simulink model "FixedWing"  (R2024b)
settings: Solver=VariableStepAuto  StartTime=0.0  StopTime=10.0  RelTol=1e-3
undefined symbols (not defined in the file): AirSpeed, Height, RollAngle
libraries: simulink_extras x3, uavalgslib x1
settings Model: Creator=shiva  LastModifiedBy=shiva

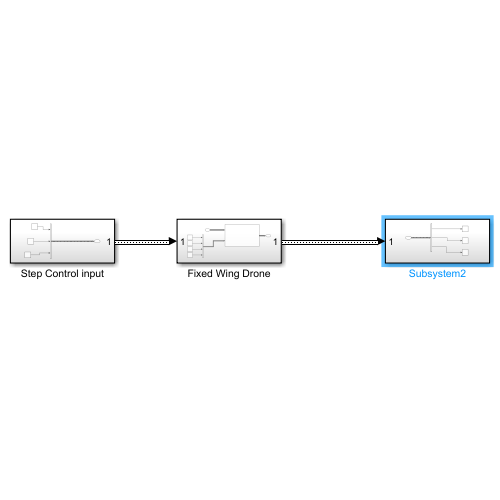
[thumbnail: Simulink's stored preview of the top-level diagram]
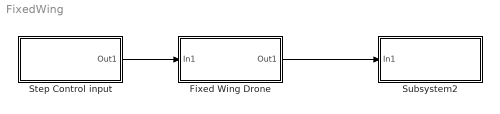
== system FixedWing ==
  Fixed Wing Drone : Subsystem
  Step Control input : Subsystem
  Subsystem2 : Subsystem
  wires:
  Step Control input/1(Out1) -> Fixed Wing Drone/1(In1)
  Fixed Wing Drone/1(Out1) -> Subsystem2/1(In1)

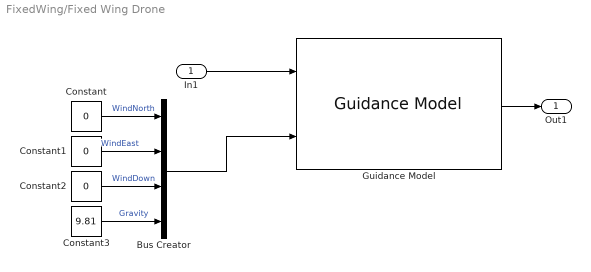
== system FixedWing/Fixed Wing Drone ==
  In1 : Inport
  Bus Creator : BusCreator  Inputs=4  OutDataTypeStr=Bus: FixedWingGuidanceEnvironmentBus  NonVirtualBus=on
  Constant : Constant  Value=0
  Constant1 : Constant  Value=0
  Constant2 : Constant  Value=0
  Constant3 : Constant  Value=9.81
  Guidance Model : uavalgslib/Guidance Model  ModelType=FixedWingGuidance  SpecifiedDataType=double  SimulateUsing=Interpreted execution  InitialWorldPositionMultirotor=[0; 0; 0]  InitialWorldVelocityMultirotor=[0; 0; 0]  InitialEulerZYXMultirotor=[0; 0; 0]  InitialBodyAngularRateRPYMultirotor=[0; 0; 0]  InitialThrustMultirotor=0  InitialNorthFixedWing=0  InitialEastFixedWing=0  InitialHeightFixedWing=0  InitialAirSpeedFixedWing=0  InitialHeadingAngleFixedWing=0  InitialFlightPathAngleFixedWing=0  InitialRollAngleFixedWing=0  InitialRollAngleRateFixedWing=0  PDRollMultirotor=[3402.97,116.67]  PDPitchMultirotor=[3402.97, 116.67]  PYawRateMultirotor=1950  PThrustMultirotor=3900  MassMultirotor=0.1  PHeightFixedWing=3.9  PHeadingAngleFixedWing=3.9  PFlightPathAngleFixedWing=39  PDRollFixedWing=[3402.97, 116.67]  PAirSpeedFixedWing=1  FlightPathAngleLimitsFixedWing=[-pi/2, pi/2]  StateBusName='FixedWingGuidanceStateBus'  ControlBusName='FixedWingGuidanceControlBus'  EnvironmentBusName='FixedWingGuidanceEnvironmentBus'  DataType=double
  Out1 : Outport
  wires:
  Guidance Model/1 -> Out1/1
  In1/1 -> Guidance Model/1
  Bus Creator/1 -> Guidance Model/2
  Constant/1 -> Bus Creator/1  "WindNorth"
  Constant1/1 -> Bus Creator/2  "WindEast"
  Constant2/1 -> Bus Creator/3  "WindDown"
  Constant3/1 -> Bus Creator/4  "Gravity"

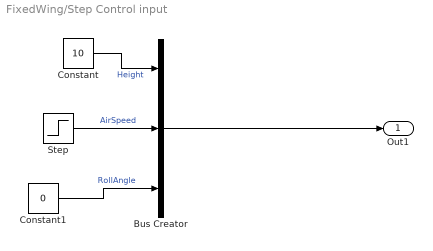
== system FixedWing/Step Control input ==
  Bus Creator : BusCreator  Inputs=Height,AirSpeed,RollAngle  OutDataTypeStr=Bus: FixedWingGuidanceControlBus  NonVirtualBus=on
  Constant : Constant  Value=10
  Constant1 : Constant  Value=0
  Step : Step  SampleTime=0
  Out1 : Outport
  wires:
  Bus Creator/1 -> Out1/1
  Constant/1 -> Bus Creator/1  "Height"
  Step/1 -> Bus Creator/2  "AirSpeed"
  Constant1/1 -> Bus Creator/3  "RollAngle"

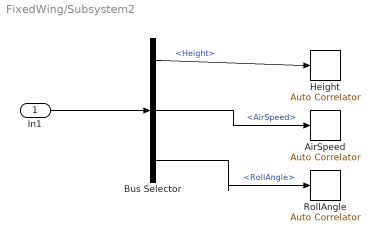
== system FixedWing/Subsystem2 ==
  In1 : Inport
  AirSpeed : simulink_extras/Additional Sinks/Auto Correlator  npts=100  HowOften=1  sampleT=0.1
  Bus Selector : BusSelector  OutputSignals=Height,AirSpeed,RollAngle
  Height : simulink_extras/Additional Sinks/Auto Correlator  npts=100  HowOften=1  sampleT=0.1
  RollAngle : simulink_extras/Additional Sinks/Auto Correlator  npts=100  HowOften=1  sampleT=0.1
  wires:
  In1/1 -> Bus Selector/1
  Bus Selector/3 -> RollAngle/1  "<RollAngle>"
  Bus Selector/2 -> AirSpeed/1  "<AirSpeed>"
  Bus Selector/1 -> Height/1  "<Height>"
